simulink library "ddm"  (R2021b)
settings: Solver=VariableStepAuto  StartTime=0.0  StopTime=10.0  RelTol=1e-3
undefined symbols (not defined in the file or in its folder): ENUM_ADASACCSTA_ERROR, ENUM_ADASACCSTA_OFF, ENUM_ADASACCSTA_STANDBY, ENUM_ADASISASTA_OFF, ENUM_ALLOWMOV_ALLOWREADY, ENUM_APS, ENUM_BRKSTA_ERROR, ENUM_BRKSTA_OFF, ENUM_BRKSTA_ON, ENUM_BRKSW_INVALID, ENUM_BRKSW_OFF, ENUM_BRKSW_ON, ENUM_CHGPREACTERRSTA_OBCPRE, ENUM_DCDCFAULTSTA_ANYFAULTLV1, ENUM_DCDCFAULTSTA_ANYFAULTLV2, ENUM_DRIVETRAIN_AWD, ENUM_DRIVETRAIN_FWD, ENUM_DRIVETRAIN_RWD, ENUM_DRSEATSTA_INVALID, ENUM_EDUDRTSTA_NORMAL, ENUM_EPBSTA_APPLIED, ENUM_EPBSTA_RELEASED, ENUM_HVBATTREADYPRE_READY, ENUM_MCUWARN_LV0, ENUM_MCUWARN_LV1, ENUM_MCUWARN_LV2, ENUM_MCUWARN_LV3, ENUM_MCUWARN_NOERROR, ENUM_OBCFAULTSTA_ANYFAULT, ENUM_PAS_R2F2, ENUM_PDFAULT_BATTPDFAIL, ENUM_PDFAULT_DCDCDISABLE, ENUM_PDFAULT_MCUDISABLE, ENUM_PDFAULT_MCUDISCHRG, ENUM_POWERSTA_OFF, ENUM_POWERSTA_ON, ENUM_POWERSTA_READY, ENUM_POWERSTA_STANDBY, ENUM_PRESSINDI_LOW, ENUM_PUFAULT_BATTUPFAIL, ENUM_PUFAULT_DCDCENABLEFAIL, ENUM_PUFAULT_PRECHRGCHKFAIL, ENUM_PUFAULT_SAFETYCHKFAIL, ENUM_PUSTATE_COMPLETED, ENUM_PWRSTASW_OFF, ENUM_PWRSTASW_OFFA, ENUM_PWRSTASW_OFFCHVCHRG, ENUM_PWRSTASW_OFFCLVCHRG, ENUM_PWRSTASW_ON, ENUM_PWRSTASW_ONHVCHRG, ENUM_PWRSTASW_READY, ENUM_PWRSTASW_STANDBY, ENUM_RANGESTA_12IN, ENUM_SHIFTCOMMAND_D, ENUM_SHIFTCOMMAND_N, ENUM_SHIFTCOMMAND_P, ENUM_SHIFTCOMMAND_R, ENUM_VEHMALFUNLV_2ND, ENUM_VEHMALFUNLV_3RD, ENUM_VEHMALFUNLV_4TH ... (+835)
libraries: hcu_lib x750, $bdroot x12, simulink x5
(part 28 of 28)

== system ddm/DDM/DDM/PMM/LV/Initial LV battery voltage too low/SR_Latch1 ==
  set : Inport
  reset : Inport  Port=2
  Logical Operator : Logic  AllPortsSameDT=off  OutDataTypeStr=boolean
  Logical Operator1 : Logic  Operator=NOT  AllPortsSameDT=off  OutDataTypeStr=boolean
  Switch1 : Switch  Criteria=u2 ~= 0  Threshold=0.5
      settings: AttributesFormatString=<Criteria=%<Criteria>>
  Switch2 : Switch  Criteria=u2 ~= 0  Threshold=0.5
      settings: AttributesFormatString=<Criteria=%<Criteria>>
  Unit Delay : UnitDelay  SampleTime=-1  HasFrameUpgradeWarning=on
  latched : Outport
  wires:
  Logical Operator1/1 -> Switch2/1, Logical Operator/2
  Logical Operator/1 -> Switch1/2
  Switch2/1 -> Switch1/3
  Unit Delay/1 -> Switch2/3
  reset/1 -> Logical Operator1/1, Switch2/2
  set/1 -> Logical Operator/1, Switch1/1
  Switch1/1 -> latched/1, Unit Delay/1

== system ddm/DDM/DDM/PMM/LV/LV power supply voltage too high/SR_Latch1 ==
  set : Inport
  reset : Inport  Port=2
  Logical Operator : Logic  AllPortsSameDT=off  OutDataTypeStr=boolean
  Logical Operator1 : Logic  Operator=NOT  AllPortsSameDT=off  OutDataTypeStr=boolean
  Switch1 : Switch  Criteria=u2 ~= 0  Threshold=0.5
      settings: AttributesFormatString=<Criteria=%<Criteria>>
  Switch2 : Switch  Criteria=u2 ~= 0  Threshold=0.5
      settings: AttributesFormatString=<Criteria=%<Criteria>>
  Unit Delay : UnitDelay  SampleTime=-1  HasFrameUpgradeWarning=on
  latched : Outport
  wires:
  Logical Operator1/1 -> Switch2/1, Logical Operator/2
  Logical Operator/1 -> Switch1/2
  Switch2/1 -> Switch1/3
  Unit Delay/1 -> Switch2/3
  reset/1 -> Logical Operator1/1, Switch2/2
  set/1 -> Logical Operator/1, Switch1/1
  Switch1/1 -> latched/1, Unit Delay/1

== system ddm/DDM/DDM/PMM/LV/LV power supply voltage too low/SR_Latch1 ==
  set : Inport
  reset : Inport  Port=2
  Logical Operator : Logic  AllPortsSameDT=off  OutDataTypeStr=boolean
  Logical Operator1 : Logic  Operator=NOT  AllPortsSameDT=off  OutDataTypeStr=boolean
  Switch1 : Switch  Criteria=u2 ~= 0  Threshold=0.5
      settings: AttributesFormatString=<Criteria=%<Criteria>>
  Switch2 : Switch  Criteria=u2 ~= 0  Threshold=0.5
      settings: AttributesFormatString=<Criteria=%<Criteria>>
  Unit Delay : UnitDelay  SampleTime=-1  HasFrameUpgradeWarning=on
  latched : Outport
  wires:
  Logical Operator1/1 -> Switch2/1, Logical Operator/2
  Logical Operator/1 -> Switch1/2
  Switch2/1 -> Switch1/3
  Unit Delay/1 -> Switch2/3
  reset/1 -> Logical Operator1/1, Switch2/2
  set/1 -> Logical Operator/1, Switch1/1
  Switch1/1 -> latched/1, Unit Delay/1

== system ddm/DDM/DDM/PMM/SW failure/Driver seat switch failure/SR_Latch3 ==
  set : Inport
  reset : Inport  Port=2
  Logical Operator : Logic  AllPortsSameDT=off  OutDataTypeStr=boolean
  Logical Operator1 : Logic  Operator=NOT  AllPortsSameDT=off  OutDataTypeStr=boolean
  Switch1 : Switch  Criteria=u2 ~= 0  Threshold=0.5
      settings: AttributesFormatString=<Criteria=%<Criteria>>
  Switch2 : Switch  Criteria=u2 ~= 0  Threshold=0.5
      settings: AttributesFormatString=<Criteria=%<Criteria>>
  Unit Delay : UnitDelay  SampleTime=-1  HasFrameUpgradeWarning=on
  latched : Outport
  wires:
  Logical Operator1/1 -> Switch2/1, Logical Operator/2
  Logical Operator/1 -> Switch1/2
  Switch2/1 -> Switch1/3
  Unit Delay/1 -> Switch2/3
  reset/1 -> Logical Operator1/1, Switch2/2
  set/1 -> Logical Operator/1, Switch1/1
  Switch1/1 -> latched/1, Unit Delay/1

== system ddm/DDM/DDM/PMM/SW failure/Driver seat switch failure/Subsystem ==
  In1 : Inport
  Trigger : TriggerPort  VariantControl=Variant  PortDimensions=1
  Constant15 : Constant  Value=KDDM_DrStSW_s
  Logical Operator3 : Logic  Operator=NOT  AllPortsSameDT=off  OutDataTypeStr=boolean
  Relational Operator3 : RelationalOperator  Operator=<=  OutDataTypeStr=boolean  RndMeth=Simplest
  SR_Latch1 : hcu_lib/Basic_Blocks/SR_Latch
  Fault_flg : Outport
  wires:
  Relational Operator3/1 -> Logical Operator3/1, SR_Latch1/1
  Constant15/1 -> Relational Operator3/2
  In1/1 -> Relational Operator3/1
  SR_Latch1/1 -> Fault_flg/1
  Logical Operator3/1 -> SR_Latch1/2

== system ddm/DDM/DDM/PMM/power up and power down/BMS HV relay closed fail/SR_Latch1 ==
  set : Inport
  reset : Inport  Port=2
  Logical Operator : Logic  AllPortsSameDT=off  OutDataTypeStr=boolean
  Logical Operator1 : Logic  Operator=NOT  AllPortsSameDT=off  OutDataTypeStr=boolean
  Switch1 : Switch  Criteria=u2 ~= 0  Threshold=0.5
      settings: AttributesFormatString=<Criteria=%<Criteria>>
  Switch2 : Switch  Criteria=u2 ~= 0  Threshold=0.5
      settings: AttributesFormatString=<Criteria=%<Criteria>>
  Unit Delay : UnitDelay  SampleTime=-1  HasFrameUpgradeWarning=on
  latched : Outport
  wires:
  Logical Operator1/1 -> Switch2/1, Logical Operator/2
  Logical Operator/1 -> Switch1/2
  Switch2/1 -> Switch1/3
  Unit Delay/1 -> Switch2/3
  reset/1 -> Logical Operator1/1, Switch2/2
  set/1 -> Logical Operator/1, Switch1/1
  Switch1/1 -> latched/1, Unit Delay/1

== system ddm/DDM/DDM/PMM/power up and power down/BMS HV relay opened fail/SR_Latch1 ==
  set : Inport
  reset : Inport  Port=2
  Logical Operator : Logic  AllPortsSameDT=off  OutDataTypeStr=boolean
  Logical Operator1 : Logic  Operator=NOT  AllPortsSameDT=off  OutDataTypeStr=boolean
  Switch1 : Switch  Criteria=u2 ~= 0  Threshold=0.5
      settings: AttributesFormatString=<Criteria=%<Criteria>>
  Switch2 : Switch  Criteria=u2 ~= 0  Threshold=0.5
      settings: AttributesFormatString=<Criteria=%<Criteria>>
  Unit Delay : UnitDelay  SampleTime=-1  HasFrameUpgradeWarning=on
  latched : Outport
  wires:
  Switch1/1 -> Unit Delay/1, latched/1
  set/1 -> Switch1/1, Logical Operator/1
  reset/1 -> Switch2/2, Logical Operator1/1
  Unit Delay/1 -> Switch2/3
  Switch2/1 -> Switch1/3
  Logical Operator/1 -> Switch1/2
  Logical Operator1/1 -> Logical Operator/2, Switch2/1

== system ddm/DDM/DDM/PMM/power up and power down/BMS ready fail/SR_Latch1 ==
  set : Inport
  reset : Inport  Port=2
  Logical Operator : Logic  AllPortsSameDT=off  OutDataTypeStr=boolean
  Logical Operator1 : Logic  Operator=NOT  AllPortsSameDT=off  OutDataTypeStr=boolean
  Switch1 : Switch  Criteria=u2 ~= 0  Threshold=0.5
      settings: AttributesFormatString=<Criteria=%<Criteria>>
  Switch2 : Switch  Criteria=u2 ~= 0  Threshold=0.5
      settings: AttributesFormatString=<Criteria=%<Criteria>>
  Unit Delay : UnitDelay  SampleTime=-1  HasFrameUpgradeWarning=on
  latched : Outport
  wires:
  Switch1/1 -> Unit Delay/1, latched/1
  set/1 -> Switch1/1, Logical Operator/1
  reset/1 -> Switch2/2, Logical Operator1/1
  Unit Delay/1 -> Switch2/3
  Switch2/1 -> Switch1/3
  Logical Operator/1 -> Switch1/2
  Logical Operator1/1 -> Logical Operator/2, Switch2/1

== system ddm/DDM/DDM/PMM/power up and power down/DCDC disable fail/SR_Latch1 ==
  set : Inport
  reset : Inport  Port=2
  Logical Operator : Logic  AllPortsSameDT=off  OutDataTypeStr=boolean
  Logical Operator1 : Logic  Operator=NOT  AllPortsSameDT=off  OutDataTypeStr=boolean
  Switch1 : Switch  Criteria=u2 ~= 0  Threshold=0.5
      settings: AttributesFormatString=<Criteria=%<Criteria>>
  Switch2 : Switch  Criteria=u2 ~= 0  Threshold=0.5
      settings: AttributesFormatString=<Criteria=%<Criteria>>
  Unit Delay : UnitDelay  SampleTime=-1  HasFrameUpgradeWarning=on
  latched : Outport
  wires:
  Switch1/1 -> Unit Delay/1, latched/1
  set/1 -> Switch1/1, Logical Operator/1
  reset/1 -> Switch2/2, Logical Operator1/1
  Unit Delay/1 -> Switch2/3
  Switch2/1 -> Switch1/3
  Logical Operator/1 -> Switch1/2
  Logical Operator1/1 -> Logical Operator/2, Switch2/1

== system ddm/DDM/DDM/PMM/power up and power down/DCDC enable fail/SR_Latch1 ==
  set : Inport
  reset : Inport  Port=2
  Logical Operator : Logic  AllPortsSameDT=off  OutDataTypeStr=boolean
  Logical Operator1 : Logic  Operator=NOT  AllPortsSameDT=off  OutDataTypeStr=boolean
  Switch1 : Switch  Criteria=u2 ~= 0  Threshold=0.5
      settings: AttributesFormatString=<Criteria=%<Criteria>>
  Switch2 : Switch  Criteria=u2 ~= 0  Threshold=0.5
      settings: AttributesFormatString=<Criteria=%<Criteria>>
  Unit Delay : UnitDelay  SampleTime=-1  HasFrameUpgradeWarning=on
  latched : Outport
  wires:
  Logical Operator1/1 -> Switch2/1, Logical Operator/2
  Logical Operator/1 -> Switch1/2
  Switch2/1 -> Switch1/3
  Unit Delay/1 -> Switch2/3
  reset/1 -> Logical Operator1/1, Switch2/2
  set/1 -> Logical Operator/1, Switch1/1
  Switch1/1 -> latched/1, Unit Delay/1

== system ddm/DDM/DDM/PMM/power up and power down/DCDC ready for precharge fail/SR_Latch1 ==
  set : Inport
  reset : Inport  Port=2
  Logical Operator : Logic  AllPortsSameDT=off  OutDataTypeStr=boolean
  Logical Operator1 : Logic  Operator=NOT  AllPortsSameDT=off  OutDataTypeStr=boolean
  Switch1 : Switch  Criteria=u2 ~= 0  Threshold=0.5
      settings: AttributesFormatString=<Criteria=%<Criteria>>
  Switch2 : Switch  Criteria=u2 ~= 0  Threshold=0.5
      settings: AttributesFormatString=<Criteria=%<Criteria>>
  Unit Delay : UnitDelay  SampleTime=-1  HasFrameUpgradeWarning=on
  latched : Outport
  wires:
  Logical Operator1/1 -> Switch2/1, Logical Operator/2
  Logical Operator/1 -> Switch1/2
  Switch2/1 -> Switch1/3
  Unit Delay/1 -> Switch2/3
  reset/1 -> Logical Operator1/1, Switch2/2
  set/1 -> Logical Operator/1, Switch1/1
  Switch1/1 -> latched/1, Unit Delay/1

== system ddm/DDM/DDM/PMM/power up and power down/HVB ready for precharge fail/SR_Latch1 ==
  set : Inport
  reset : Inport  Port=2
  Logical Operator : Logic  AllPortsSameDT=off  OutDataTypeStr=boolean
  Logical Operator1 : Logic  Operator=NOT  AllPortsSameDT=off  OutDataTypeStr=boolean
  Switch1 : Switch  Criteria=u2 ~= 0  Threshold=0.5
      settings: AttributesFormatString=<Criteria=%<Criteria>>
  Switch2 : Switch  Criteria=u2 ~= 0  Threshold=0.5
      settings: AttributesFormatString=<Criteria=%<Criteria>>
  Unit Delay : UnitDelay  SampleTime=-1  HasFrameUpgradeWarning=on
  latched : Outport
  wires:
  Logical Operator1/1 -> Switch2/1, Logical Operator/2
  Logical Operator/1 -> Switch1/2
  Switch2/1 -> Switch1/3
  Unit Delay/1 -> Switch2/3
  reset/1 -> Logical Operator1/1, Switch2/2
  set/1 -> Logical Operator/1, Switch1/1
  Switch1/1 -> latched/1, Unit Delay/1

== system ddm/DDM/DDM/PMM/power up and power down/High level system safety check fail/SR_Latch1 ==
  set : Inport
  reset : Inport  Port=2
  Logical Operator : Logic  AllPortsSameDT=off  OutDataTypeStr=boolean
  Logical Operator1 : Logic  Operator=NOT  AllPortsSameDT=off  OutDataTypeStr=boolean
  Switch1 : Switch  Criteria=u2 ~= 0  Threshold=0.5
      settings: AttributesFormatString=<Criteria=%<Criteria>>
  Switch2 : Switch  Criteria=u2 ~= 0  Threshold=0.5
      settings: AttributesFormatString=<Criteria=%<Criteria>>
  Unit Delay : UnitDelay  SampleTime=-1  HasFrameUpgradeWarning=on
  latched : Outport
  wires:
  Switch1/1 -> Unit Delay/1, latched/1
  set/1 -> Switch1/1, Logical Operator/1
  reset/1 -> Switch2/2, Logical Operator1/1
  Unit Delay/1 -> Switch2/3
  Switch2/1 -> Switch1/3
  Logical Operator/1 -> Switch1/2
  Logical Operator1/1 -> Logical Operator/2, Switch2/1

== system ddm/DDM/DDM/PMM/power up and power down/MCU active discharge fail/SR_Latch1 ==
  set : Inport
  reset : Inport  Port=2
  Logical Operator : Logic  AllPortsSameDT=off  OutDataTypeStr=boolean
  Logical Operator1 : Logic  Operator=NOT  AllPortsSameDT=off  OutDataTypeStr=boolean
  Switch1 : Switch  Criteria=u2 ~= 0  Threshold=0.5
      settings: AttributesFormatString=<Criteria=%<Criteria>>
  Switch2 : Switch  Criteria=u2 ~= 0  Threshold=0.5
      settings: AttributesFormatString=<Criteria=%<Criteria>>
  Unit Delay : UnitDelay  SampleTime=-1  HasFrameUpgradeWarning=on
  latched : Outport
  wires:
  Switch1/1 -> Unit Delay/1, latched/1
  set/1 -> Switch1/1, Logical Operator/1
  reset/1 -> Switch2/2, Logical Operator1/1
  Unit Delay/1 -> Switch2/3
  Switch2/1 -> Switch1/3
  Logical Operator/1 -> Switch1/2
  Logical Operator1/1 -> Logical Operator/2, Switch2/1

== system ddm/DDM/DDM/PMM/power up and power down/MCU disable fail/SR_Latch1 ==
  set : Inport
  reset : Inport  Port=2
  Logical Operator : Logic  AllPortsSameDT=off  OutDataTypeStr=boolean
  Logical Operator1 : Logic  Operator=NOT  AllPortsSameDT=off  OutDataTypeStr=boolean
  Switch1 : Switch  Criteria=u2 ~= 0  Threshold=0.5
      settings: AttributesFormatString=<Criteria=%<Criteria>>
  Switch2 : Switch  Criteria=u2 ~= 0  Threshold=0.5
      settings: AttributesFormatString=<Criteria=%<Criteria>>
  Unit Delay : UnitDelay  SampleTime=-1  HasFrameUpgradeWarning=on
  latched : Outport
  wires:
  Switch1/1 -> Unit Delay/1, latched/1
  set/1 -> Switch1/1, Logical Operator/1
  reset/1 -> Switch2/2, Logical Operator1/1
  Unit Delay/1 -> Switch2/3
  Switch2/1 -> Switch1/3
  Logical Operator/1 -> Switch1/2
  Logical Operator1/1 -> Logical Operator/2, Switch2/1

== system ddm/DDM/DDM/PMM/power up and power down/MCU ready for precharge fail/SR_Latch1 ==
  set : Inport
  reset : Inport  Port=2
  Logical Operator : Logic  AllPortsSameDT=off  OutDataTypeStr=boolean
  Logical Operator1 : Logic  Operator=NOT  AllPortsSameDT=off  OutDataTypeStr=boolean
  Switch1 : Switch  Criteria=u2 ~= 0  Threshold=0.5
      settings: AttributesFormatString=<Criteria=%<Criteria>>
  Switch2 : Switch  Criteria=u2 ~= 0  Threshold=0.5
      settings: AttributesFormatString=<Criteria=%<Criteria>>
  Unit Delay : UnitDelay  SampleTime=-1  HasFrameUpgradeWarning=on
  latched : Outport
  wires:
  Logical Operator1/1 -> Switch2/1, Logical Operator/2
  Logical Operator/1 -> Switch1/2
  Switch2/1 -> Switch1/3
  Unit Delay/1 -> Switch2/3
  reset/1 -> Logical Operator1/1, Switch2/2
  set/1 -> Logical Operator/1, Switch1/1
  Switch1/1 -> latched/1, Unit Delay/1

== system ddm/DDM/DDM/PMM/power up and power down/Mid level system safety check fail/SR_Latch1 ==
  set : Inport
  reset : Inport  Port=2
  Logical Operator : Logic  AllPortsSameDT=off  OutDataTypeStr=boolean
  Logical Operator1 : Logic  Operator=NOT  AllPortsSameDT=off  OutDataTypeStr=boolean
  Switch1 : Switch  Criteria=u2 ~= 0  Threshold=0.5
      settings: AttributesFormatString=<Criteria=%<Criteria>>
  Switch2 : Switch  Criteria=u2 ~= 0  Threshold=0.5
      settings: AttributesFormatString=<Criteria=%<Criteria>>
  Unit Delay : UnitDelay  SampleTime=-1  HasFrameUpgradeWarning=on
  latched : Outport
  wires:
  Switch1/1 -> Unit Delay/1, latched/1
  set/1 -> Switch1/1, Logical Operator/1
  reset/1 -> Switch2/2, Logical Operator1/1
  Unit Delay/1 -> Switch2/3
  Switch2/1 -> Switch1/3
  Logical Operator/1 -> Switch1/2
  Logical Operator1/1 -> Logical Operator/2, Switch2/1

== system ddm/DDM/DDM/PMM/power up and power down/OBC ready for precharge fail/SR_Latch1 ==
  set : Inport
  reset : Inport  Port=2
  Logical Operator : Logic  AllPortsSameDT=off  OutDataTypeStr=boolean
  Logical Operator1 : Logic  Operator=NOT  AllPortsSameDT=off  OutDataTypeStr=boolean
  Switch1 : Switch  Criteria=u2 ~= 0  Threshold=0.5
      settings: AttributesFormatString=<Criteria=%<Criteria>>
  Switch2 : Switch  Criteria=u2 ~= 0  Threshold=0.5
      settings: AttributesFormatString=<Criteria=%<Criteria>>
  Unit Delay : UnitDelay  SampleTime=-1  HasFrameUpgradeWarning=on
  latched : Outport
  wires:
  Switch1/1 -> Unit Delay/1, latched/1
  set/1 -> Switch1/1, Logical Operator/1
  reset/1 -> Switch2/2, Logical Operator1/1
  Unit Delay/1 -> Switch2/3
  Switch2/1 -> Switch1/3
  Logical Operator/1 -> Switch1/2
  Logical Operator1/1 -> Logical Operator/2, Switch2/1

== system ddm/DDM/DDM/VMC_DDM/FCM4/FCM4 Rolling Count Error /SR_Latch1 ==
  set : Inport
  reset : Inport  Port=2
  Logical Operator : Logic  AllPortsSameDT=off  OutDataTypeStr=boolean
  Logical Operator1 : Logic  Operator=NOT  AllPortsSameDT=off  OutDataTypeStr=boolean
  Switch1 : Switch  Criteria=u2 ~= 0  Threshold=0.5
      settings: AttributesFormatString=<Criteria=%<Criteria>>
  Switch2 : Switch  Criteria=u2 ~= 0  Threshold=0.5
      settings: AttributesFormatString=<Criteria=%<Criteria>>
  Unit Delay : UnitDelay  SampleTime=-1  HasFrameUpgradeWarning=on
  latched : Outport
  wires:
  Logical Operator1/1 -> Switch2/1, Logical Operator/2
  Logical Operator/1 -> Switch1/2
  Switch2/1 -> Switch1/3
  Unit Delay/1 -> Switch2/3
  reset/1 -> Logical Operator1/1, Switch2/2
  set/1 -> Logical Operator/1, Switch1/1
  Switch1/1 -> latched/1, Unit Delay/1

== system ddm/DDM/DDM/VMC_DDM/FCM4/FCM4 Rolling Count Error /Test Detection Criteria ==
  trigger : Inport
  Ts : Inport  Port=2
  KDDM_xxxDTC_cnt : Inport  Port=3
  KDDM_xxxDetTO_s : Inport  Port=4
  Constant35 : Constant  Value=ZERO_INT
  Data Type Conversion : DataTypeConversion  OutDataTypeStr=single
  Data Type Conversion1 : DataTypeConversion  OutDataTypeStr=uint16
  Detect Increase : simulink/Logic and Bit Operations/Detect Increase  vinit=0.0  OutDataTypeStr=boolean
  Equal9 : RelationalOperator  Operator===  OutDataTypeStr=boolean  RndMeth=Simplest
  Gain : Gain  Gain=KXX2XX  RndMeth=Round
  Gain1 : Gain  Gain=KXX2XX
  Logical Operator19 : Logic  AllPortsSameDT=off  OutDataTypeStr=boolean
  Logical Operator3 : Logic  Operator=NOT  AllPortsSameDT=off  OutDataTypeStr=boolean
  ModMath : Subsystem  mask(Count){}
      mask help: Counter function.
      mask Display:
      | fprintf('ModMath');
      | port_label('output', 1, 'Remainder');
      | port_label('input', 1, 'Dividend');
      | port_label('input', 2, 'Divisor');
  Product : Product
  Rounding Function : Rounding  Operator=round
  Rounding Function1 : Rounding  Operator=round
  Timer : Subsystem  mask(Timer){}
      mask help: Timer funcion.
  VDDM_xxxDet_flg : Outport
  wires:
  Rounding Function1/1 -> ModMath/2(Divisor)
  Rounding Function/1 -> ModMath/1(Dividend)
  Data Type Conversion1/1 -> Equal9/1
  Gain1/1 -> Rounding Function1/1
  Gain/1 -> Rounding Function/1
  Detect Increase/1 -> VDDM_xxxDet_flg/1
  ModMath/1(Remainder) -> Data Type Conversion1/1
  KDDM_xxxDTC_cnt/1 -> Data Type Conversion/1
  KDDM_xxxDetTO_s/1 -> Product/1, [KDDM_xxxDetTO_s]
  Data Type Conversion/1 -> Product/2
  Product/1 -> Timer/4(max_time)
  Ts/1 -> Timer/3(Ts)
  Timer/1(time) -> Gain/1
  Logical Operator3/1 -> Timer/2(reset)
  Equal9/1 -> Logical Operator19/2
  [KDDM_xxxDetTO_s] -> Gain1/1
  trigger/1 -> Logical Operator3/1, Logical Operator19/1, Timer/1(trigger)
  Logical Operator19/1 -> Detect Increase/1
  Constant35/1 -> Equal9/2

== system ddm/DDM/DDM/VMC_DDM/FCM4/FCM4 Rolling Count Error /Timer1 ==
  note: /* output signal type is single */
  trigger : Inport
  reset : Inport  Port=2
  Ts : Inport  Port=3
  max_time : Inport  Port=4
  Constant1 : Constant  Value=ZERO_FLOAT  OutDataTypeStr=single
  MinMax : MinMax  Inputs=2
  Subtract2 : Sum
  Switch1 : Switch  Criteria=u2 ~= 0
      settings: AttributesFormatString=<%<Criteria>>
  Switch2 : Switch  Criteria=u2 ~= 0
      settings: AttributesFormatString=<%<Criteria>>
  Unit Delay1 : UnitDelay  SampleTime=-1  HasFrameUpgradeWarning=on
      settings: AttributesFormatString=<initial = %<X0>>
  time : Outport
  wires:
  [last_time] -> Subtract2/1
  max_time/1 -> MinMax/1
  Unit Delay1/1 -> [last_time], Switch1/3
  MinMax/1 -> Unit Delay1/1, time/1
  Switch2/1 -> MinMax/2
  Ts/1 -> Subtract2/2
  Switch1/1 -> Switch2/3
  Constant1/1 -> Switch1/1
  reset/1 -> Switch1/2
  trigger/1 -> Switch2/2
  Subtract2/1 -> Switch2/1

== system ddm/DDM/DDM/VMC_DDM/FCM5/FCM5 Rolling Count Error /SR_Latch1 ==
  set : Inport
  reset : Inport  Port=2
  Logical Operator : Logic  AllPortsSameDT=off  OutDataTypeStr=boolean
  Logical Operator1 : Logic  Operator=NOT  AllPortsSameDT=off  OutDataTypeStr=boolean
  Switch1 : Switch  Criteria=u2 ~= 0  Threshold=0.5
      settings: AttributesFormatString=<Criteria=%<Criteria>>
  Switch2 : Switch  Criteria=u2 ~= 0  Threshold=0.5
      settings: AttributesFormatString=<Criteria=%<Criteria>>
  Unit Delay : UnitDelay  SampleTime=-1  HasFrameUpgradeWarning=on
  latched : Outport
  wires:
  Logical Operator1/1 -> Switch2/1, Logical Operator/2
  Logical Operator/1 -> Switch1/2
  Switch2/1 -> Switch1/3
  Unit Delay/1 -> Switch2/3
  reset/1 -> Logical Operator1/1, Switch2/2
  set/1 -> Logical Operator/1, Switch1/1
  Switch1/1 -> latched/1, Unit Delay/1

== system ddm/DDM/DDM/VMC_DDM/FCM5/FCM5 Rolling Count Error /Test Detection Criteria ==
  trigger : Inport
  Ts : Inport  Port=2
  KDDM_xxxDTC_cnt : Inport  Port=3
  KDDM_xxxDetTO_s : Inport  Port=4
  Constant35 : Constant  Value=ZERO_INT
  Data Type Conversion : DataTypeConversion  OutDataTypeStr=single
  Data Type Conversion1 : DataTypeConversion  OutDataTypeStr=uint16
  Detect Increase : simulink/Logic and Bit Operations/Detect Increase  vinit=0.0  OutDataTypeStr=boolean
  Equal9 : RelationalOperator  Operator===  OutDataTypeStr=boolean  RndMeth=Simplest
  Gain : Gain  Gain=KXX2XX  RndMeth=Round
  Gain1 : Gain  Gain=KXX2XX
  Logical Operator19 : Logic  AllPortsSameDT=off  OutDataTypeStr=boolean
  Logical Operator3 : Logic  Operator=NOT  AllPortsSameDT=off  OutDataTypeStr=boolean
  ModMath : Subsystem  mask(Count){}
      mask help: Counter function.
      mask Display:
      | fprintf('ModMath');
      | port_label('output', 1, 'Remainder');
      | port_label('input', 1, 'Dividend');
      | port_label('input', 2, 'Divisor');
  Product : Product
  Rounding Function : Rounding  Operator=round
  Rounding Function1 : Rounding  Operator=round
  Timer : Subsystem  mask(Timer){}
      mask help: Timer funcion.
  VDDM_xxxDet_flg : Outport
  wires:
  Rounding Function1/1 -> ModMath/2(Divisor)
  Rounding Function/1 -> ModMath/1(Dividend)
  Data Type Conversion1/1 -> Equal9/1
  Gain1/1 -> Rounding Function1/1
  Gain/1 -> Rounding Function/1
  Detect Increase/1 -> VDDM_xxxDet_flg/1
  ModMath/1(Remainder) -> Data Type Conversion1/1
  KDDM_xxxDTC_cnt/1 -> Data Type Conversion/1
  KDDM_xxxDetTO_s/1 -> Product/1, [KDDM_xxxDetTO_s]
  Data Type Conversion/1 -> Product/2
  Product/1 -> Timer/4(max_time)
  Ts/1 -> Timer/3(Ts)
  Timer/1(time) -> Gain/1
  Logical Operator3/1 -> Timer/2(reset)
  Equal9/1 -> Logical Operator19/2
  [KDDM_xxxDetTO_s] -> Gain1/1
  trigger/1 -> Logical Operator3/1, Logical Operator19/1, Timer/1(trigger)
  Logical Operator19/1 -> Detect Increase/1
  Constant35/1 -> Equal9/2

== system ddm/DDM/DDM/VMC_DDM/FCM5/FCM5 Rolling Count Error /Timer1 ==
  note: /* output signal type is single */
  trigger : Inport
  reset : Inport  Port=2
  Ts : Inport  Port=3
  max_time : Inport  Port=4
  Constant1 : Constant  Value=ZERO_FLOAT  OutDataTypeStr=single
  MinMax : MinMax  Inputs=2
  Subtract2 : Sum
  Switch1 : Switch  Criteria=u2 ~= 0
      settings: AttributesFormatString=<%<Criteria>>
  Switch2 : Switch  Criteria=u2 ~= 0
      settings: AttributesFormatString=<%<Criteria>>
  Unit Delay1 : UnitDelay  SampleTime=-1  HasFrameUpgradeWarning=on
      settings: AttributesFormatString=<initial = %<X0>>
  time : Outport
  wires:
  [last_time] -> Subtract2/1
  max_time/1 -> MinMax/1
  Unit Delay1/1 -> [last_time], Switch1/3
  MinMax/1 -> Unit Delay1/1, time/1
  Switch2/1 -> MinMax/2
  Ts/1 -> Subtract2/2
  Switch1/1 -> Switch2/3
  Constant1/1 -> Switch1/1
  reset/1 -> Switch1/2
  trigger/1 -> Switch2/2
  Subtract2/1 -> Switch2/1

== system ddm/DDM/DDM/VMC_DDM/FCM4/FCM4 Rolling Count Error /Test Detection Criteria/ModMath ==
  Dividend : Inport
  Divisor : Inport  Port=2
  Abs : Abs
  Constant : Constant  Value=eps
  Data Type Conversion : DataTypeConversion
  Data Type Conversion1 : DataTypeConversion
  Data Type Conversion2 : DataTypeConversion  OutDataTypeStr=single
  Display : Display
      settings: Format=long_e
  Divide : Product  Inputs=*/
  Equal : RelationalOperator  Operator=<=  OutDataTypeStr=boolean  RndMeth=Simplest
  Floor : Rounding
  Minus : Sum  Inputs=+-
  Product : Product
  Switch : Switch  Criteria=u2 > Threshold
  Remainder : Outport
  wires:
  [Divisor] -> Abs/1
  Product/1 -> Data Type Conversion/1
  Divide/1 -> Data Type Conversion2/1
  [Divisor] -> Product/2
  Abs/1 -> Equal/1
  [Divisor] -> Divide/2
  Data Type Conversion1/1 -> Product/1
  Floor/1 -> Data Type Conversion1/1
  Dividend/1 -> [Dividend]
  [Dividend] -> Minus/1
  Data Type Conversion/1 -> Minus/2
  Data Type Conversion2/1 -> Floor/1
  Minus/1 -> Switch/3, Display/1
  [Dividend] -> Switch/1
  Switch/1 -> Remainder/1
  [Dividend] -> Divide/1
  Constant/1 -> Equal/2
  Equal/1 -> Switch/2
  Divisor/1 -> [Divisor]

== system ddm/DDM/DDM/VMC_DDM/FCM4/FCM4 Rolling Count Error /Test Detection Criteria/Timer ==
  note: /* output signal type is single */
  trigger : Inport
  reset : Inport  Port=2
  Ts : Inport  Port=3
  max_time : Inport  Port=4
  Constant1 : Constant  Value=ZERO_FLOAT  OutDataTypeStr=single
  MinMax : MinMax  Inputs=2
  Subtract2 : Sum
  Switch1 : Switch  Criteria=u2 ~= 0
      settings: AttributesFormatString=<%<Criteria>>
  Switch2 : Switch  Criteria=u2 ~= 0
      settings: AttributesFormatString=<%<Criteria>>
  Unit Delay1 : UnitDelay  SampleTime=-1  HasFrameUpgradeWarning=on
      settings: AttributesFormatString=<initial = %<X0>>
  time : Outport
  wires:
  [last_time] -> Subtract2/1
  max_time/1 -> MinMax/1
  Unit Delay1/1 -> [last_time], Switch1/3
  MinMax/1 -> Unit Delay1/1, time/1
  Switch2/1 -> MinMax/2
  Ts/1 -> Subtract2/2
  Switch1/1 -> Switch2/3
  Constant1/1 -> Switch1/1
  reset/1 -> Switch1/2
  trigger/1 -> Switch2/2
  Subtract2/1 -> Switch2/1

== system ddm/DDM/DDM/VMC_DDM/FCM5/FCM5 Rolling Count Error /Test Detection Criteria/ModMath ==
  Dividend : Inport
  Divisor : Inport  Port=2
  Abs : Abs
  Constant : Constant  Value=eps
  Data Type Conversion : DataTypeConversion
  Data Type Conversion1 : DataTypeConversion
  Data Type Conversion2 : DataTypeConversion  OutDataTypeStr=single
  Display : Display
      settings: Format=long_e
  Divide : Product  Inputs=*/
  Equal : RelationalOperator  Operator=<=  OutDataTypeStr=boolean  RndMeth=Simplest
  Floor : Rounding
  Minus : Sum  Inputs=+-
  Product : Product
  Switch : Switch  Criteria=u2 > Threshold
  Remainder : Outport
  wires:
  [Divisor] -> Abs/1
  Product/1 -> Data Type Conversion/1
  Divide/1 -> Data Type Conversion2/1
  [Divisor] -> Product/2
  Abs/1 -> Equal/1
  [Divisor] -> Divide/2
  Data Type Conversion1/1 -> Product/1
  Floor/1 -> Data Type Conversion1/1
  Dividend/1 -> [Dividend]
  [Dividend] -> Minus/1
  Data Type Conversion/1 -> Minus/2
  Data Type Conversion2/1 -> Floor/1
  Minus/1 -> Switch/3, Display/1
  [Dividend] -> Switch/1
  Switch/1 -> Remainder/1
  [Dividend] -> Divide/1
  Constant/1 -> Equal/2
  Equal/1 -> Switch/2
  Divisor/1 -> [Divisor]

== system ddm/DDM/DDM/VMC_DDM/FCM5/FCM5 Rolling Count Error /Test Detection Criteria/Timer ==
  note: /* output signal type is single */
  trigger : Inport
  reset : Inport  Port=2
  Ts : Inport  Port=3
  max_time : Inport  Port=4
  Constant1 : Constant  Value=ZERO_FLOAT  OutDataTypeStr=single
  MinMax : MinMax  Inputs=2
  Subtract2 : Sum
  Switch1 : Switch  Criteria=u2 ~= 0
      settings: AttributesFormatString=<%<Criteria>>
  Switch2 : Switch  Criteria=u2 ~= 0
      settings: AttributesFormatString=<%<Criteria>>
  Unit Delay1 : UnitDelay  SampleTime=-1  HasFrameUpgradeWarning=on
      settings: AttributesFormatString=<initial = %<X0>>
  time : Outport
  wires:
  [last_time] -> Subtract2/1
  max_time/1 -> MinMax/1
  Unit Delay1/1 -> [last_time], Switch1/3
  MinMax/1 -> Unit Delay1/1, time/1
  Switch2/1 -> MinMax/2
  Ts/1 -> Subtract2/2
  Switch1/1 -> Switch2/3
  Constant1/1 -> Switch1/1
  reset/1 -> Switch1/2
  trigger/1 -> Switch2/2
  Subtract2/1 -> Switch2/1

== stateflow chart ddm/DDM/DDM/Chart ==
  (default) -> (junction 3)
  (junction 3) -> (junction 5) [order 1] : [VDDM_Lv4ErrCFS_flg || ...
      |  ZoneFrMalfunLevel_enum == ENUM_ZONEMALFUNLV_4TH || ...
      |  ZoneDrMalfunLevel_enum == ENUM_ZONEMALFUNLV_4TH]
  (junction 3) -> (junction 9) [order 2]
  (junction 5) -> (junction 18) : {VDDM_VehMalfunLevel_enum = 4;
      |  %Warning_lamp = 1;
      |  %IVI_popup = 4;
      |  VDDM_limphome_enum = 4;
      |  VDDM_EmergencyPwrDown_flg = TRUE;}
  (junction 9) -> (junction 14) [order 1] : [VDDM_C3BMS1RCCFS_flg || ...
      |  VDDM_C3BMS1CSCFS_flg || ...
      |  VDDM_C3BMS1LCCFS_flg || ...
      |  VDDM_Lv3ErrCFS_flg || ...
      |  VDDM_HVB4PreCFS_flg || ...
      |  VDDM_MCU4PreCFS_flg || ...
      |  VDDM_DCDC4PreCFS_flg || ...
      |  VDDM_HVRlyCloCFS_flg || ...
      |  VDDM_BMSRdyCFS_flg || ...
      |  VDDM_DCDCEnaCFS_flg || ...
      |  VDDM_HiLvSaChkCFS_flg || ...
      |  VDDM_MidLvSaChkCFS_flg || ...
      |  VDDM_HVRlyOpCFS_flg || ...
      |  VDDM_MCUActCFS_flg || ...
      |  VDDM_MCUF1NoComCFS_flg || ...
      |  VDDM_MCUR1NoComCFS_flg || ...
      |  VDDM_MCUF1RCErrCFS_flg || ...
      |  VDDM_MCUR1RCErrCFS_flg || ...
      |  VDDM_MCUF1CSErrCFS_flg || ...
      |  VDDM_MCUR1CSErrCFS_flg || ...
      |  ZoneFrMalfunLevel_enum == ENUM_ZONEMALFUNLV_3RD || ...
      |  ZoneDrMalfunLevel_enum == ENUM_ZONEMALFUNLV_3RD]
  (junction 9) -> (junction 22) [order 2]
  (junction 14) -> (junction 19) : {VDDM_VehMalfunLevel_enum = 3;
      |  %Warning_lamp = 1;
      |  %IVI_popup = 3;
      |  VDDM_limphome_enum = 3;
      |  VDDM_EmergencyPwrDown_flg = FALSE;}
  (junction 22) -> (junction 24) [order 1] : [VDDM_C3BMS6RCCFS_flg || ...
      |  VDDM_C3BMS6CSCFS_flg || ...
      |  VDDM_C3BMS6LCCFS_flg || ...
      |  VDDM_C3CCU1RCCFS_flg || ...
      |  VDDM_C3CCU1CSCFS_flg || ...
      |  VDDM_C3CCU1LCCFS_flg || ...
      |  VDDM_C3CCU2RCCFS_flg || ...
      |  VDDM_C3CCU2CSCFS_flg || ...
      |  VDDM_C3CCU2LCCFS_flg || ...
      |  VDDM_Lv2ErrCFS_flg || ...
      |  VDDM_IniLVLoCFS_flg || ...
      |  VDDM_LVSupLoCFS_flg || ...
      |  VDDM_LVSupHiCFS_flg || ...
      |  VDDM_BrkSWNoBacCFS_flg || ...
      |  VDDM_ESC7NoComCFS_flg || ...
      |  VDDM_ESC1NoComCFS_flg || ...
      |  VDDM_ESC5NoComCFS_flg || ...
      |  VDDM_ESC7RCErrCFS_flg || ...
      |  VDDM_ESC1RCErrCFS_flg || ...
      |  VDDM_ESC5RCErrCFS_flg || ...
      | VDDM_ESC7CSErrCFS_flg || ...
      |  VDDM_ESC1CSErrCFS_flg || ...
      |  VDDM_ESC5CSErrCFS_flg || ...
      |  VDDM_5vAPS1PwrErrCFS_flg || ...
      |  VDDM_5vAPS2PwrErrCFS_flg || ...
      |  VDDM_5vAPS1OoCFS_flg || ...
      |  VDDM_5vAPS2OoCFS_flg || ...
      |  VDDM_APS1SigOoRCFS_flg || ...
      |  VDDM_APS2SigOoRCFS_flg || ...
      |  VDDM_APSCorrErrCFS_flg || ...
      |  ZoneFrMalfunLevel_enum == ENUM_ZONEMALFUNLV_2ND || ...
      |  ZoneDrMalfunLevel_enum == ENUM_ZONEMALFUNLV_2ND]
  (junction 22) -> (junction 29) [order 2]
  (junction 24) -> (junction 26) : {VDDM_VehMalfunLevel_enum = 2;
      |  %Warning_lamp = 1;
      |  %IVI_popup = 2;
      |  VDDM_limphome_enum = 2;
      |  VDDM_EmergencyPwrDown_flg = FALSE;}
  (junction 29) -> (junction 31) [order 1] : [VDDM_C1ABM1RCCFS_flg || ...
      |  VDDM_C1ABM1CSCFS_flg || ...
      |  VDDM_C1ABM1LCCFS_flg || ...
      |  VDDM_Lv1ErrCFS_flg || ...
      |  VDDM_MCUDisCFS_flg || ...
      |  VDDM_DCDCDisCFS_flg || ...
      |  VDDM_OBC4PreCFS_flg || ...
      |  VDDM_BrkSWErrCFS_flg || ...
      |  VDDM_DrStSWCFS_flg || ...
      |  VDDM_FLDoorSWCFS_flg || ...
      |  VDDM_FRDoorSWCFS_flg || ...
      |  VDDM_RLDoorSWCFS_flg || ...
      |  VDDM_RRDoorSWCFS_flg || ...
      |  VDDM_HoodSWCFS_flg || ...
      |  VDDM_TailgaSWCFS_flg || ...
      |  VDDM_KeyAuthCFS_flg || ...
      |  VDDM_LVChFrqCFS_flg || ...
      |  VDDM_ONtoRdyCFS_flg || ...
      |  VDDM_Shifter1NoComCFS_flg || ...
      |  VDDM_Shifter1RCErrCFS_flg || ...
      |  VDDM_Shifter1CSErrCFS_flg || ...
      |  VDDM_EPBLockTOCFS_flg || ...
      |  VDDM_EPBUnlockTOCFS_flg || ...
      |  ZoneFrMalfunLevel_enum == ENUM_ZONEMALFUNLV_1ST || ...
      |  ZoneDrMalfunLevel_enum == ENUM_ZONEMALFUNLV_1ST]
  (junction 29) -> (junction 36) [order 2] : {VDDM_VehMalfunLevel_enum = 0;
      |  %Warning_lamp = 0;
      |  %IVI_popup = 0;
      |  VDDM_limphome_enum = 0;
      |  VDDM_EmergencyPwrDown_flg = FALSE;}
  (junction 31) -> (junction 33) : {VDDM_VehMalfunLevel_enum = 1;
      |  %Warning_lamp = 0;
      |  %IVI_popup = 0;
      |  VDDM_limphome_enum = 0;
      |  VDDM_EmergencyPwrDown_flg = FALSE;}
  (junction 33) -> (junction 36)
  (junction 26) -> (junction 33)
  (junction 19) -> (junction 26)
  (junction 18) -> (junction 19)
  data: VDDM_Lv4ErrCFS_flg input; VDDM_5vAPS1OoCFS_flg input; VDDM_5vAPS1PwrErrCFS_flg input; VDDM_5vAPS2OoCFS_flg input; VDDM_5vAPS2PwrErrCFS_flg input; VDDM_BMSRdyCFS_flg input; VDDM_BrkSWErrCFS_flg input; VDDM_BrkSWNoBacCFS_flg input; VDDM_C1ABM1CSCFS_flg input; VDDM_C1ABM1LCCFS_flg input; VDDM_C1ABM1RCCFS_flg input; VDDM_C3BMS1CSCFS_flg input; VDDM_C3BMS1LCCFS_flg input; VDDM_C3BMS1RCCFS_flg input; VDDM_C3BMS6CSCFS_flg input; VDDM_C3BMS6LCCFS_flg input; VDDM_C3BMS6RCCFS_flg input; VDDM_C3CCU1CSCFS_flg input; VDDM_C3CCU1LCCFS_flg input; VDDM_C3CCU1RCCFS_flg input; VDDM_C3CCU2CSCFS_flg input; VDDM_C3CCU2LCCFS_flg input; VDDM_C3CCU2RCCFS_flg input; VDDM_DCDC4PreCFS_flg input; VDDM_DCDCDisCFS_flg input; VDDM_DCDCEnaCFS_flg input; VDDM_DrStSWCFS_flg input; VDDM_EPBLockTOCFS_flg input; VDDM_EPBUnlockTOCFS_flg input; VDDM_ESC1CSErrCFS_flg input; VDDM_ESC1NoComCFS_flg input; VDDM_ESC1RCErrCFS_flg input; VDDM_ESC5CSErrCFS_flg input; VDDM_ESC5NoComCFS_flg input; VDDM_ESC5RCErrCFS_flg input; VDDM_ESC7CSErrCFS_flg input; VDDM_ESC7NoComCFS_flg input; VDDM_ESC7RCErrCFS_flg input; VDDM_FLDoorSWCFS_flg input; VDDM_FRDoorSWCFS_flg input; VDDM_HVB4PreCFS_flg input; VDDM_HVRlyCloCFS_flg input; VDDM_HVRlyOpCFS_flg input; VDDM_HiLvSaChkCFS_flg input; VDDM_IniLVLoCFS_flg input; VDDM_KeyAuthCFS_flg input; VDDM_LVChFrqCFS_flg input; VDDM_LVSupHiCFS_flg input; VDDM_LVSupLoCFS_flg input; VDDM_Lv1ErrCFS_flg input; VDDM_Lv2ErrCFS_flg input; VDDM_Lv3ErrCFS_flg input; VDDM_MCU4PreCFS_flg input; VDDM_MCUActCFS_flg input; VDDM_MCUDisCFS_flg input; VDDM_MCUF1CSErrCFS_flg input; VDDM_MCUF1NoComCFS_flg input; VDDM_MCUF1RCErrCFS_flg input; VDDM_MCUR1CSErrCFS_flg input; VDDM_MCUR1NoComCFS_flg input; VDDM_MCUR1RCErrCFS_flg input; VDDM_MidLvSaChkCFS_flg input; VDDM_OBC4PreCFS_flg input; VDDM_ONtoRdyCFS_flg input; VDDM_RLDoorSWCFS_flg input; VDDM_RRDoorSWCFS_flg input; VDDM_Shifter1CSErrCFS_flg input; VDDM_Shifter1NoComCFS_flg input; VDDM_Shifter1RCErrCFS_flg input; VDDM_VehMalfunLevel_enum output uint8; VDDM_EmergencyPwrDown_flg output boolean; VDDM_limphome_enum output uint8; VDDM_HoodSWCFS_flg input; VDDM_TailgaSWCFS_flg input; ZoneDrMalfunLevel_enum input; ZoneFrMalfunLevel_enum input; ENUM_ZONEMALFUNLV_1ST parameter; ENUM_ZONEMALFUNLV_2ND parameter; ENUM_ZONEMALFUNLV_3RD parameter; ENUM_ZONEMALFUNLV_4TH parameter; FALSE parameter; TRUE parameter; VDDM_APS1SigOoRCFS_flg input; VDDM_APS2SigOoRCFS_flg input; VDDM_APSCorrErrCFS_flg input
